simulink model "yaw_lineal"  (R2015a)
settings: Solver=ode45  StartTime=0.0  StopTime=68.0  RelTol=1e-3
values from neighbouring files (symbols this model uses):
  Kyaw = 4*Kpsi*Km/Izz    (= 8.61428571429)    [Parametros.m]
  ty = 0.0002251891410    (= 0.000225189141)    [Parametros.m]
libraries: simulink x5
settings Model: Creator=simaqtel  LastModifiedBy=Eduardo

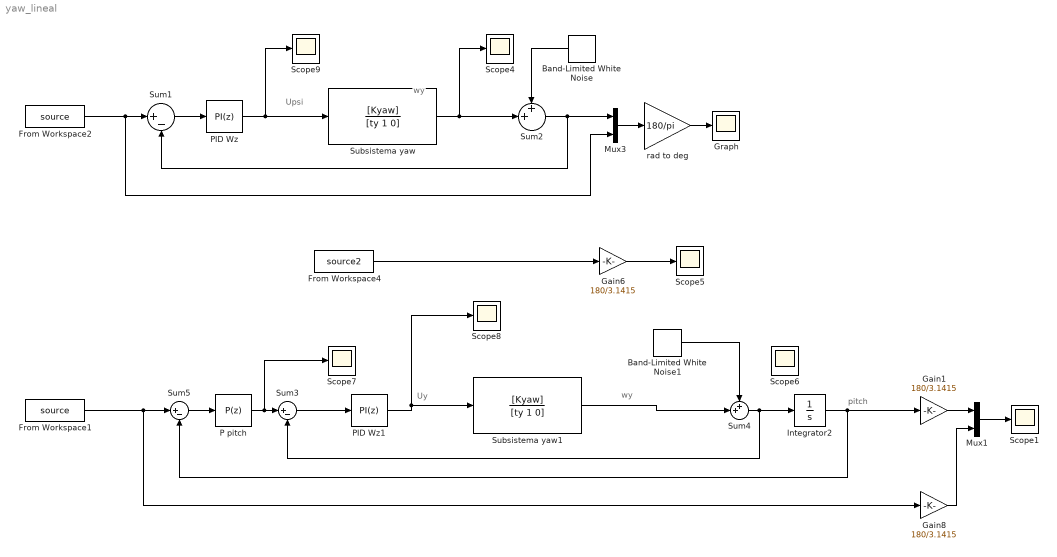
== system yaw_lineal ==
  note: pitch
  note: wy
  note: Upsi
  note: wy
  note: Uy
  Band-Limited White Noise : simulink/Sources/Band-Limited White Noise  Cov=[0.000001]  Ts=0.01  seed=[23341]
  Band-Limited White Noise1 : simulink/Sources/Band-Limited White Noise  Cov=[0.000001]  Ts=0.01  seed=[23341]
  From Workspace1 : FromWorkspace  VariableName=source  SampleTime=0.01
  From Workspace2 : FromWorkspace  VariableName=source  SampleTime=0.01
  From Workspace4 : FromWorkspace  VariableName=source2  SampleTime=0.01
  Gain1 : Gain  Gain=180/3.1415
  Gain6 : Gain  Gain=180/3.1415
  Gain8 : Gain  Gain=180/3.1415
  Graph : Scope
      settings: SaveName=ScopeData3
  Integrator2 : Integrator
  Mux1 : Mux  Inputs=2
  Mux3 : Mux  Inputs=2
  P pitch : simulink/Continuous/PID Controller  Controller=P  TimeDomain=Discrete-time  SampleTime=0.01  IntegratorMethod=Forward Euler  FilterMethod=Forward Euler  Form=Parallel  UseFilter=off  ControllerParametersSource=internal  P=6.15  I=0.5  D=0.05  N=20.2444442041031  InitialConditionSource=internal  InitialConditionForIntegrator=0  InitialConditionForFilter=0  ExternalReset=none  LimitOutput=off  UpperSaturationLimit=3  LowerSaturationLimit=-3  LinearizeAsGain=on  AntiWindupMode=none  Kb=1  TrackingMode=off  Kt=1  PParamMin=[]  PParamMax=[]  IParamMin=[]  IParamMax=[]  DParamMin=[]  DParamMax=[]  NParamMin=[]  NParamMax=[]  KbParamMin=[]  KbParamMax=[]  KtParamMin=[]  KtParamMax=[]  POutMin=[]  POutMax=[]  IOutMin=[]  IOutMax=[]  DOutMin=[]  DOutMax=[]  NOutMin=[]  NOutMax=[]  KbOutMin=[]  KbOutMax=[]  KtOutMin=[]  KtOutMax=[]  IntegratorOutMin=[]  IntegratorOutMax=[]  FilterOutMin=[]  FilterOutMax=[]  SumOutMin=[]  SumOutMax=[]  SumI1OutMin=[]  SumI1OutMax=[]  SumI2OutMin=[]  SumI2OutMax=[]  SumI3OutMin=[]  SumI3OutMax=[]  SumDOutMin=[]  SumDOutMax=[]  SaturationOutMin=[]  SaturationOutMax=[]  IntegratorContinuousStateAttributes=''  IntegratorStateMustResolveToSignalObject=off  IntegratorRTWStateStorageClass=Auto  FilterContinuousStateAttributes=''  FilterStateMustResolveToSignalObject=off  FilterRTWStateStorageClass=Auto  DifferentiatorICPrevScaledInput=0  DifferentiatorOutMin=[]  DifferentiatorOutMax=[]
  PID Wz : simulink/Continuous/PID Controller  Controller=PI  TimeDomain=Discrete-time  SampleTime=0.01  IntegratorMethod=Forward Euler  FilterMethod=Forward Euler  Form=Ideal  UseFilter=on  ControllerParametersSource=internal  P=2.01  I=0.142  D=0.0957187049121133  N=189.58120119176  InitialConditionSource=internal  InitialConditionForIntegrator=0  InitialConditionForFilter=0  ExternalReset=none  LimitOutput=on  UpperSaturationLimit=1  LowerSaturationLimit=-1  LinearizeAsGain=on  AntiWindupMode=back-calculation  Kb=0.1  TrackingMode=off  Kt=1  PParamMin=[]  PParamMax=[]  IParamMin=[]  IParamMax=[]  DParamMin=[]  DParamMax=[]  NParamMin=[]  NParamMax=[]  KbParamMin=[]  KbParamMax=[]  KtParamMin=[]  KtParamMax=[]  POutMin=[]  POutMax=[]  IOutMin=[]  IOutMax=[]  DOutMin=[]  DOutMax=[]  NOutMin=[]  NOutMax=[]  KbOutMin=[]  KbOutMax=[]  KtOutMin=[]  KtOutMax=[]  IntegratorOutMin=[]  IntegratorOutMax=[]  FilterOutMin=[]  FilterOutMax=[]  SumOutMin=[]  SumOutMax=[]  SumI1OutMin=[]  SumI1OutMax=[]  SumI2OutMin=[]  SumI2OutMax=[]  SumI3OutMin=[]  SumI3OutMax=[]  SumDOutMin=[]  SumDOutMax=[]  SaturationOutMin=[]  SaturationOutMax=[]  IntegratorContinuousStateAttributes=''  IntegratorStateMustResolveToSignalObject=off  IntegratorRTWStateStorageClass=Auto  FilterContinuousStateAttributes=''  FilterStateMustResolveToSignalObject=off  FilterRTWStateStorageClass=Auto  DifferentiatorICPrevScaledInput=0  DifferentiatorOutMin=[]  DifferentiatorOutMax=[]
  PID Wz1 : simulink/Continuous/PID Controller  Controller=PI  TimeDomain=Discrete-time  SampleTime=0.01  IntegratorMethod=Forward Euler  FilterMethod=Forward Euler  Form=Ideal  UseFilter=on  ControllerParametersSource=internal  P=2.92191286824416  I=0.206490361247336  D=0.0957187049121133  N=189.58120119176  InitialConditionSource=internal  InitialConditionForIntegrator=0  InitialConditionForFilter=0  ExternalReset=none  LimitOutput=on  UpperSaturationLimit=1  LowerSaturationLimit=-1  LinearizeAsGain=on  AntiWindupMode=none  Kb=0.2  TrackingMode=off  Kt=1  PParamMin=[]  PParamMax=[]  IParamMin=[]  IParamMax=[]  DParamMin=[]  DParamMax=[]  NParamMin=[]  NParamMax=[]  KbParamMin=[]  KbParamMax=[]  KtParamMin=[]  KtParamMax=[]  POutMin=[]  POutMax=[]  IOutMin=[]  IOutMax=[]  DOutMin=[]  DOutMax=[]  NOutMin=[]  NOutMax=[]  KbOutMin=[]  KbOutMax=[]  KtOutMin=[]  KtOutMax=[]  IntegratorOutMin=[]  IntegratorOutMax=[]  FilterOutMin=[]  FilterOutMax=[]  SumOutMin=[]  SumOutMax=[]  SumI1OutMin=[]  SumI1OutMax=[]  SumI2OutMin=[]  SumI2OutMax=[]  SumI3OutMin=[]  SumI3OutMax=[]  SumDOutMin=[]  SumDOutMax=[]  SaturationOutMin=[]  SaturationOutMax=[]  IntegratorContinuousStateAttributes=''  IntegratorStateMustResolveToSignalObject=off  IntegratorRTWStateStorageClass=Auto  FilterContinuousStateAttributes=''  FilterStateMustResolveToSignalObject=off  FilterRTWStateStorageClass=Auto  DifferentiatorICPrevScaledInput=0  DifferentiatorOutMin=[]  DifferentiatorOutMax=[]
  Scope{1,4..9} (7 alike) : Scope
      Scope1 settings: TimeRange=1.085807108091082  YMin=-1.321354166666669  YMax=18.16197916666667
      Scope4 settings: SaveName=ScopeData4
      Scope5 settings: SaveName=ScopeData5
      Scope7 settings: SaveName=ScopeData6
      Scope8 settings: SaveName=ScopeData7
      Scope9 settings: SaveName=ScopeData8
  Subsistema yaw : TransferFcn  Numerator=[Kyaw]  Denominator=[ty 1 0]
  Subsistema yaw1 : TransferFcn  Numerator=[Kyaw]  Denominator=[ty 1 0]
  Sum1 : Sum  Inputs=|+-
  Sum2 : Sum  Inputs=++|
  Sum3 : Sum  Inputs=|+-
  Sum4 : Sum  Inputs=++|
  Sum5 : Sum  Inputs=|+-
  rad to deg : Gain  Gain=180/pi
  wires:
  Sum1/1 -> PID Wz/1
  From Workspace4/1 -> Gain6/1
  Sum2/1 -> Sum1/2, Mux3/1
  Subsistema yaw/1 -> Scope4/1, Sum2/2
  Band-Limited White Noise/1 -> Sum2/1
  Gain6/1 -> Scope5/1
  Mux1/1 -> Scope1/1
  Gain1/1 -> Mux1/1
  Sum4/1 -> Integrator2/1, Sum3/2
  Band-Limited White Noise1/1 -> Sum4/1
  Gain8/1 -> Mux1/2
  P pitch/1 -> Scope7/1, Sum3/1
  Sum5/1 -> P pitch/1
  From Workspace1/1 -> Gain8/1, Sum5/1
  Integrator2/1 -> Gain1/1, Sum5/2
  From Workspace2/1 -> Mux3/2, Sum1/1
  PID Wz/1 -> Scope9/1, Subsistema yaw/1
  PID Wz1/1 -> Subsistema yaw1/1, Scope8/1
  Sum3/1 -> PID Wz1/1
  rad to deg/1 -> Graph/1
  Mux3/1 -> rad to deg/1
  Subsistema yaw1/1 -> Sum4/2
